simulink model "torque_structure"  (R2024b)
settings: Solver=FixedStepDiscrete  StartTime=0.0  StopTime=10.0  FixedStep=Ts  RelTol=1e-3
values from neighbouring files (symbols this model uses):
  g = 9.81    [main_data_vehicle.m]
  L = 1.55    [main_data_vehicle.m]
  lf = L*fr    (= 0.7905)    [main_data_vehicle.m]
  lr = L-lf    (= 0.7595)    [main_data_vehicle.m]
  Re = 0.259    [main_data_vehicle.m]
  TC = 1    [main_data_vehicle.m]
  TV = 1    [main_data_vehicle.m]
undefined symbols (not defined in the file or in its folder): DiscIntNeverNeededParam
libraries: simulink_extras x4, simulink x4, slpidlib x3
settings Model: Creator=marti  LastModifiedBy=marti

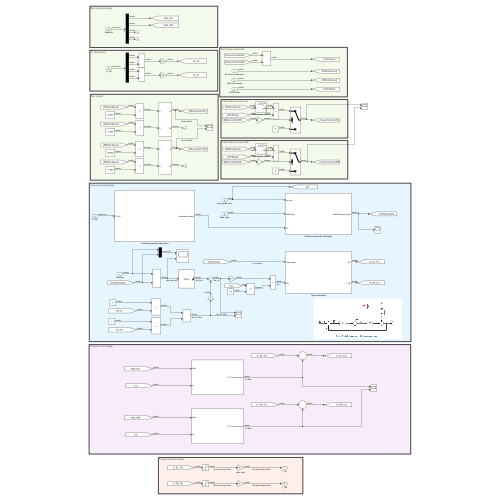
[thumbnail: Simulink's stored preview of the top-level diagram]
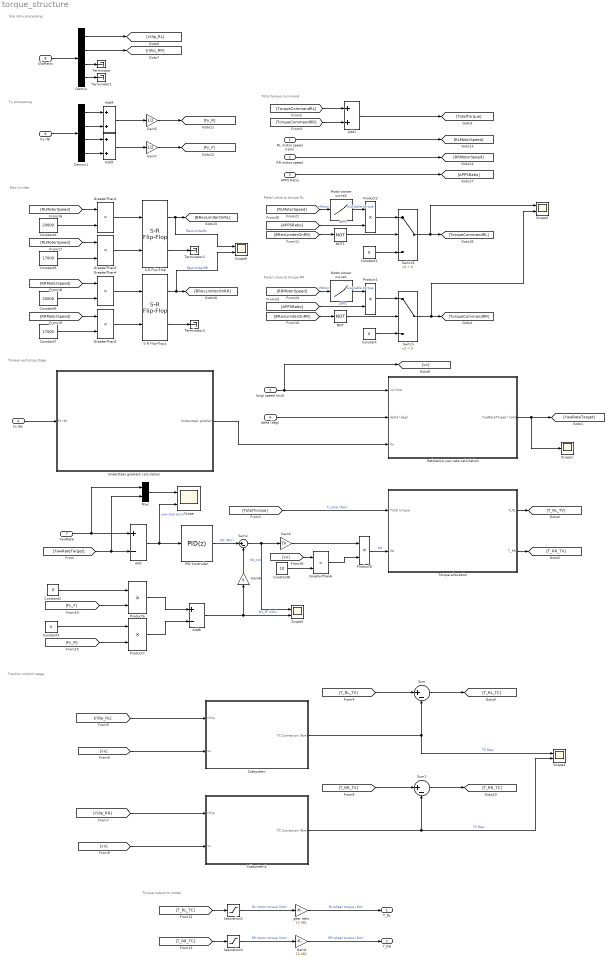
== system torque_structure ==
  note: Rev Limiter
  note: Fy processing
  note: Torque output to model
  note: Traction control stage
  note: Slip ratio processing
  note: Torque vectoring stage
  note: Total torque command
  note: Pedal value to torque RL
  note: Pedal value to torque RR
  RL motor speed (rpm) : Inport
  RR motor speed : Inport  Port=2
  APPS Ratio : Inport  Port=3
  Fz (N) : Inport  Port=4
  longi speed (m/s) : Inport  Port=5
  delta (deg) : Inport  Port=6
  YawRate : Inport  Port=7
  SlipRatio : Inport  Port=8
  Fy (N) : Inport  Port=9
  Add : Sum  Inputs=+-
  Add1 : Sum
  Add4 : Sum
  Add5 : Sum
  Add6 : Sum  Inputs=+-
  Constant : Constant  Value=0
  Constant1 : Constant  Value=0
  Constant2 : Constant  Value=lf
  Constant3 : Constant  Value=lr
  Constant4 : Constant  Value=20000
  Constant5 : Constant  Value=17000
  Constant6 : Constant  Value=20000
  Constant7 : Constant  Value=17000
  Constant8 : Constant  Value=10
  Demux : Demux
  Demux1 : Demux
  Gain2 : Gain  Gain=TV
  Gain5 : Gain  Gain=1/2
  Gain6 : Gain  Gain=12.481
  Gain7 : Gain  Gain=1/2
  Gain8 : Gain  Gain=0
  GreaterThan2 : RelationalOperator  Operator=>  OutDataTypeStr=boolean  RndMeth=Simplest  InputSameDT=off
  GreaterThan3 : RelationalOperator  Operator=<  OutDataTypeStr=boolean  RndMeth=Simplest  InputSameDT=off
  GreaterThan4 : RelationalOperator  Operator=>  OutDataTypeStr=boolean  RndMeth=Simplest  InputSameDT=off
  GreaterThan5 : RelationalOperator  Operator=<  OutDataTypeStr=boolean  RndMeth=Simplest  InputSameDT=off
  GreaterThan6 : RelationalOperator  Operator=>  OutDataTypeStr=boolean  RndMeth=Simplest  InputSameDT=off
  Motor power curve1 : Lookup_n-D  NumberOfTableDimensions=1  BreakpointsForDimension1=[0 11500 20000 20001]  Table=[32 32 18 0]  ExtrapMethod=Clip  UseLastTableValue=on  InternalRulePriority=Speed  RndMeth=Simplest
  Motor power curve2 : Lookup_n-D  NumberOfTableDimensions=1  BreakpointsForDimension1=[0 11500 20000 20001]  Table=[32 32 18 0]  ExtrapMethod=Clip  UseLastTableValue=on  InternalRulePriority=Speed  RndMeth=Simplest
  Mux : Mux  Inputs=2
  NOT : Logic  Operator=NOT  IconShape=distinctive  AllPortsSameDT=off  OutDataTypeStr=boolean
  NOT1 : Logic  Operator=NOT  IconShape=distinctive  AllPortsSameDT=off  OutDataTypeStr=boolean
  PID Controller : slpidlib/PID Controller  Controller=PID  Form=Parallel  TimeDomain=Discrete-time  UseExternalTs=off  SampleTime=-1  IntegratorMethod=Forward Euler  FilterMethod=Forward Euler  ControllerParametersSource=internal  P=100  I=0  UseKiTs=off  D=0  UseExternalDerivativeSource=off  N=100  UseFilter=on  TunerSelectOption=Transfer Function Based (PID Tuner App)  InitialConditionSource=internal  InitialConditionForIntegrator=0  InitialConditionForFilter=0  DifferentiatorICPrevScaledInput=0  ExternalReset=none  TrackingMode=off  Kt=1  LimitOutput=on  SatLimitsSource=internal  UpperSaturationLimit=500  LowerSaturationLimit=-500  LinearizeAsGain=on  AntiWindupMode=clamping  Kb=10  LimitIntegrator=off  UpperIntegratorSaturationLimit=inf  LowerIntegratorSaturationLimit=-inf  POutMin=[]  POutMax=[]  IOutMin=[]  IOutMax=[]  DOutMin=[]  DOutMax=[]  NOutMin=[]  NOutMax=[]  SumOutMin=[]  SumOutMax=[]  SaturationOutMin=[]  SaturationOutMax=[]  PParamMin=[]  PParamMax=[]  IParamMin=[]  IParamMax=[]  DParamMin=[]  DParamMax=[]  NParamMin=[]  NParamMax=[]  KbParamMin=[]  KbParamMax=[]  KtParamMin=[]  KtParamMax=[]  KbOutMin=[]  KbOutMax=[]  KtOutMin=[]  KtOutMax=[]  IntegratorOutMin=[]  IntegratorOutMax=[]  FilterOutMin=[]  FilterOutMax=[]  SumI1OutMin=[]  SumI1OutMax=[]  SumI2OutMin=[]  SumI2OutMax=[]  SumI3OutMin=[]  SumI3OutMax=[]  SumI4OutMin=[]  SumI4OutMax=[]  SumDOutMin=[]  SumDOutMax=[]  DifferentiatorOutMin=[]  DifferentiatorOutMax=[]  FilterDiffOutCoefMin=[]  FilterDiffOutCoefMax=[]  ReciprocalOutMin=[]  ReciprocalOutMax=[]  SumDenOutMin=[]  SumDenOutMax=[]  SumNumOutMin=[]  SumNumOutMax=[]  DivideOutMin=[]  DivideOutMax=[]  UdiffTsProdOutMin=[]  UdiffTsProdOutMax=[]  NTsProdOutMin=[]  NTsProdOutMax=[]  UintegralTsProdOutMin=[]  UintegralTsProdOutMax=[]  UngainTsProdOutMin=[]  UngainTsProdOutMax=[]  ClampingZeroOutDataTypeStr=Inherit: Inherit via back propagation  ClampingZeroOutMin=[]  ClampingZeroOutMax=[]  FilterDenConstantOutDataTypeStr=Inherit: Inherit via back propagation  FilterDenConstantOutMin=[]  FilterDenConstantOutMax=[]  PCopyOutDataTypeStr=Inherit: Inherit via back propagation  PCopyOutMin=[]  PCopyOutMax=[]  NCopyOutDataTypeStr=Inherit: Inherit via back propagation  NCopyOutMin=[]  NCopyOutMax=[]  IntegratorContinuousStateAttributes=''  IntegratorStateMustResolveToSignalObject=off  IntegratorRTWStateStorageClass=Auto  FilterContinuousStateAttributes=''  FilterStateMustResolveToSignalObject=off  FilterRTWStateStorageClass=Auto  ParallelPVariant=InternalParameters  IdealPVariant=Disabled  IVariant=InternalParameters  DVariant=InternalParameters  IntegratorVariant=Discrete  SatVariant=Enabled  AWVariant=DiscClampingParallel  PCopyVariant=Disabled  TRVariant=Disabled  FdbkBlocksVariant=Forward  IdealPFdbkVariant=Disabled  SatFdbkVariant=Disabled  DerivativeFilterVariant=ForwardEulerFilter  NVariant=InternalParameters  NCopyVariant=Disabled  FilterICVariant=InternalICsFilter  IntegratorICVariant=InternalICs  ExternalResetVariant=Disabled  TRSumVariant=Passthrough  SumFdbkVariant=Disabled  SumVariant=Sum_PID  TsampFilterVariant=InternalTs  TsampNgainVariant=Passthrough  TsampIntegralVariant=Disabled_SignalSpec  ExternalSaturationOutDataTypeStr=Inherit: Same as second input  DerivativeSourceVariant=ErrorSignal  PreIntVariant=InternalPreInt
  Product{1..2,6..8} (5 alike) : Product
  Reference yaw rate calculation : Subsystem
  S-R Flip-Flop : simulink_extras/Flip Flops/S-R Flip-Flop  initial_condition=0
  S-R Flip-Flop1 : simulink_extras/Flip Flops/S-R Flip-Flop  initial_condition=0
  Saturation2 : Saturate  UpperLimit=32  LowerLimit=-32
  Saturation3 : Saturate  UpperLimit=32  LowerLimit=-32
  Scope{,2..5} (5 alike) : Scope  NumInputPorts=2
  Scope1 : Scope
  Subsystem : Subsystem
  Subsystem1 : Subsystem
  Sum : Sum  Inputs=|+-
  Sum1 : Sum  Inputs=|+-
  Sum2 : Sum  Inputs=|+-
  Switch : Switch  Criteria=u2 > Threshold  SaturateOnIntegerOverflow=off  InputSameDT=off
  Switch1 : Switch  Criteria=u2 > Threshold  SaturateOnIntegerOverflow=off  InputSameDT=off
  Terminator{,1..3} (4 alike) : Terminator
  Torque allocation : Subsystem
  Understeer gradient calculation : Subsystem
  gear ratio : Gain  Gain=12.481
  T_RL : Outport
  T_RR : Outport  Port=2
  wires:
  Fz (N)/1 -> Understeer gradient calculation/1(Fz (N))
  Understeer gradient calculation/1(Understeer gradient) -> Reference yaw rate calculation/3(Ku)
  delta (deg)/1 -> Reference yaw rate calculation/2(delta (deg))
  longi speed (m/s)/1 -> [vx], Reference yaw rate calculation/1(vx (m/s))
  Reference yaw rate calculation/1(YawRateTarget (rad/s)) -> Scope1/1, [YawRateTarget]
  YawRate/1 -> Mux/1, Add/1
  [YawRateTarget] -> Mux/2, Add/2
  Add/1 -> Scope/2, PID Controller/1  "yaw rate error"
  [TotalTorque] -> Torque allocation/1(Total torque)  "T_total (Nm)"
  [TorqueCommandRL] -> Add1/1
  [TorqueCommandRR] -> Add1/2
  Add1/1 -> [TotalTorque]
  Torque allocation/1(T_RL) -> [T_RL_TV]
  Torque allocation/2(T_RR) -> [T_RR_TV]
  SlipRatio/1 -> Demux/1
  Demux/1 -> [rSlip_RL]
  Demux/2 -> [rSlip_RR]
  Demux/3 -> Terminator/1
  Demux/4 -> Terminator1/1
  [T_RL_TV] -> Sum/1
  [T_RR_TV] -> Sum1/1
  [T_RL_TC] -> Saturation2/1
  [T_RR_TC] -> Saturation3/1
  Saturation2/1 -> gear ratio/1  "RL motor torque (Nm)"
  Saturation3/1 -> Gain6/1  "RR motor torque (Nm)"
  gear ratio/1 -> T_RL/1  "RL wheel torque (Nm)"
  Gain6/1 -> T_RR/1  "RR wheel torque (Nm)"
  Sum/1 -> [T_RL_TC]
  Sum1/1 -> [T_RR_TC]
  Mux/1 -> Scope/1
  Fy (N)/1 -> Demux1/1
  Demux1/1 -> Add4/1
  Demux1/2 -> Add4/2
  Demux1/3 -> Add5/1
  Demux1/4 -> Add5/2
  Add4/1 -> Gain5/1
  Add5/1 -> Gain7/1
  Gain5/1 -> [Fy_R]
  Gain7/1 -> [Fy_F]
  Constant2/1 -> Product6/1
  [Fy_F] -> Product6/2
  [Fy_R] -> Product7/2
  Constant3/1 -> Product7/1
  Product6/1 -> Add6/1
  Product7/1 -> Add6/2
  PID Controller/1 -> Sum2/1  "Mz (Nm)"
  Sum2/1 -> Scope2/1, Gain2/1  "Mz_tot"
  Add6/1 -> Gain8/1, Scope2/2  "Mz_FF (Nm)"
  RL motor speed (rpm)/1 -> [RLMotorSpeed]
  RR motor speed/1 -> [RRMotorSpeed]
  [RLMotorSpeed] -> GreaterThan2/1
  Constant4/1 -> GreaterThan2/2
  GreaterThan2/1 -> S-R Flip-Flop/1
  Constant5/1 -> GreaterThan3/2
  [RLMotorSpeed] -> GreaterThan3/1
  GreaterThan3/1 -> S-R Flip-Flop/2
  S-R Flip-Flop/1 -> Scope5/1, [BRevLimiterOnRL]  "RevLimiterRL"
  S-R Flip-Flop/2 -> Terminator2/1
  S-R Flip-Flop1/2 -> Terminator3/1
  S-R Flip-Flop1/1 -> Scope5/2, [BRevLimiterOnRR]  "RevLimiterRR"
  GreaterThan5/1 -> S-R Flip-Flop1/2
  [RRMotorSpeed] -> GreaterThan5/1
  Constant7/1 -> GreaterThan5/2
  GreaterThan4/1 -> S-R Flip-Flop1/1
  Constant6/1 -> GreaterThan4/2
  [RRMotorSpeed] -> GreaterThan4/1
  APPS Ratio/1 -> [APPSRatio]
  [APPSRatio] -> Product1/2  "APPS"
  Motor power curve1/1 -> Product1/1  "available torque"
  [RRMotorSpeed] -> Motor power curve1/1  "nMotor"
  [vx] -> GreaterThan6/1
  Product8/1 -> Torque allocation/2(Mz)  "Mz"
  Gain2/1 -> Product8/1
  Gain8/1 -> Sum2/2
  Constant8/1 -> GreaterThan6/2
  GreaterThan6/1 -> Product8/2
  [rSlip_RL] -> Subsystem/1(rSlip)
  [vx] -> Subsystem/2(vx)
  [vx] -> Subsystem1/2(vx)
  [rSlip_RR] -> Subsystem1/1(rSlip)
  Switch/1 -> Scope3/2, [TorqueCommandRR]
  Product1/1 -> Switch/1
  [BRevLimiterOnRR] -> NOT/1
  NOT/1 -> Switch/2
  Constant/1 -> Switch/3
  Constant1/1 -> Switch1/3
  NOT1/1 -> Switch1/2
  [BRevLimiterOnRR] -> NOT1/1
  Product2/1 -> Switch1/1
  Switch1/1 -> Scope3/1, [TorqueCommandRL]
  [RLMotorSpeed] -> Motor power curve2/1  "nMotor"
  Motor power curve2/1 -> Product2/1  "available torque"
  [APPSRatio] -> Product2/2  "APPS"
  Subsystem/1(TC Correction (Nm)) -> Scope4/1, Sum/2  "TC Raw"
  Subsystem1/1(TC Correction (Nm)) -> Scope4/2, Sum1/2  "TC Raw"

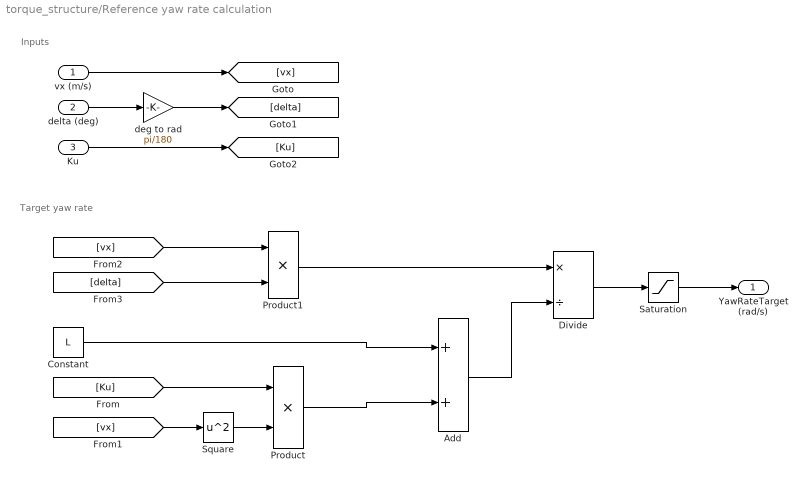
== system torque_structure/Reference yaw rate calculation ==
  note: Target yaw rate
  note: Inputs
  vx (m/s) : Inport
  delta (deg) : Inport  Port=2
  Ku : Inport  Port=3
  Add : Sum
  Constant : Constant  Value=L
  Divide : Product  Inputs=*/
  Product : Product
  Product1 : Product
  Saturation : Saturate  UpperLimit=1.5  LowerLimit=-1.5
  Square : Math  Operator=square
  deg to rad : Gain  Gain=pi/180
  YawRateTarget (rad/s) : Outport
  wires:
  vx (m/s)/1 -> [vx]
  delta (deg)/1 -> deg to rad/1
  deg to rad/1 -> [delta]
  Ku/1 -> [Ku]
  [vx] -> Square/1
  Square/1 -> Product/2
  [Ku] -> Product/1
  Product/1 -> Add/2
  Constant/1 -> Add/1
  [vx] -> Product1/1
  [delta] -> Product1/2
  Product1/1 -> Divide/1
  Add/1 -> Divide/2
  Divide/1 -> Saturation/1
  Saturation/1 -> YawRateTarget (rad/s)/1

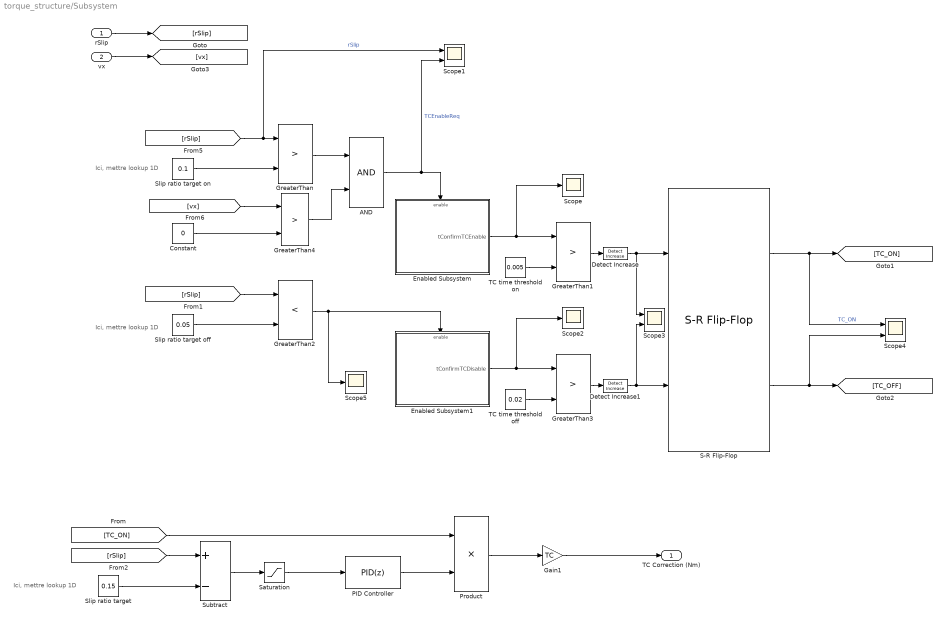
== system torque_structure/Subsystem ==
  note: Ici, mettre lookup 1D
  note: Ici, mettre lookup 1D
  note: Ici, mettre lookup 1D
  rSlip : Inport
  vx : Inport  Port=2
  AND : Logic  AllPortsSameDT=off  OutDataTypeStr=boolean
  Constant : Constant  Value=0
  Detect Increase : simulink/Logic and Bit Operations/Detect Increase  vinit=0.0  OutDataTypeStr=boolean
  Detect Increase1 : simulink/Logic and Bit Operations/Detect Increase  vinit=0.0  OutDataTypeStr=boolean
  Enabled Subsystem : Subsystem  TreatAsAtomicUnit=on
  Enabled Subsystem1 : Subsystem  TreatAsAtomicUnit=on
  Gain1 : Gain  Gain=TC
  GreaterThan{,1,3..4} (4 alike) : RelationalOperator  Operator=>  OutDataTypeStr=boolean  RndMeth=Simplest  InputSameDT=off
  GreaterThan2 : RelationalOperator  Operator=<  OutDataTypeStr=boolean  RndMeth=Simplest  InputSameDT=off
  PID Controller : slpidlib/PID Controller  Controller=PID  Form=Parallel  TimeDomain=Discrete-time  UseExternalTs=off  SampleTime=-1  IntegratorMethod=Forward Euler  FilterMethod=Forward Euler  ControllerParametersSource=internal  P=100  I=20  UseKiTs=off  D=0  UseExternalDerivativeSource=off  N=100  UseFilter=on  TunerSelectOption=Transfer Function Based (PID Tuner App)  InitialConditionSource=internal  InitialConditionForIntegrator=0  InitialConditionForFilter=0  DifferentiatorICPrevScaledInput=0  ExternalReset=none  TrackingMode=off  Kt=1  LimitOutput=on  SatLimitsSource=internal  UpperSaturationLimit=30  LowerSaturationLimit=0  LinearizeAsGain=on  AntiWindupMode=clamping  Kb=1  LimitIntegrator=off  UpperIntegratorSaturationLimit=inf  LowerIntegratorSaturationLimit=-inf  POutMin=[]  POutMax=[]  IOutMin=[]  IOutMax=[]  DOutMin=[]  DOutMax=[]  NOutMin=[]  NOutMax=[]  SumOutMin=[]  SumOutMax=[]  SaturationOutMin=[]  SaturationOutMax=[]  PParamMin=[]  PParamMax=[]  IParamMin=[]  IParamMax=[]  DParamMin=[]  DParamMax=[]  NParamMin=[]  NParamMax=[]  KbParamMin=[]  KbParamMax=[]  KtParamMin=[]  KtParamMax=[]  KbOutMin=[]  KbOutMax=[]  KtOutMin=[]  KtOutMax=[]  IntegratorOutMin=[]  IntegratorOutMax=[]  FilterOutMin=[]  FilterOutMax=[]  SumI1OutMin=[]  SumI1OutMax=[]  SumI2OutMin=[]  SumI2OutMax=[]  SumI3OutMin=[]  SumI3OutMax=[]  SumI4OutMin=[]  SumI4OutMax=[]  SumDOutMin=[]  SumDOutMax=[]  DifferentiatorOutMin=[]  DifferentiatorOutMax=[]  FilterDiffOutCoefMin=[]  FilterDiffOutCoefMax=[]  ReciprocalOutMin=[]  ReciprocalOutMax=[]  SumDenOutMin=[]  SumDenOutMax=[]  SumNumOutMin=[]  SumNumOutMax=[]  DivideOutMin=[]  DivideOutMax=[]  UdiffTsProdOutMin=[]  UdiffTsProdOutMax=[]  NTsProdOutMin=[]  NTsProdOutMax=[]  UintegralTsProdOutMin=[]  UintegralTsProdOutMax=[]  UngainTsProdOutMin=[]  UngainTsProdOutMax=[]  ClampingZeroOutDataTypeStr=Inherit: Inherit via back propagation  ClampingZeroOutMin=[]  ClampingZeroOutMax=[]  FilterDenConstantOutDataTypeStr=Inherit: Inherit via back propagation  FilterDenConstantOutMin=[]  FilterDenConstantOutMax=[]  PCopyOutDataTypeStr=Inherit: Inherit via back propagation  PCopyOutMin=[]  PCopyOutMax=[]  NCopyOutDataTypeStr=Inherit: Inherit via back propagation  NCopyOutMin=[]  NCopyOutMax=[]  IntegratorContinuousStateAttributes=''  IntegratorStateMustResolveToSignalObject=off  IntegratorRTWStateStorageClass=Auto  FilterContinuousStateAttributes=''  FilterStateMustResolveToSignalObject=off  FilterRTWStateStorageClass=Auto  ParallelPVariant=InternalParameters  IdealPVariant=Disabled  IVariant=InternalParameters  DVariant=InternalParameters  IntegratorVariant=Discrete  SatVariant=Enabled  AWVariant=DiscClampingParallel  PCopyVariant=Disabled  TRVariant=Disabled  FdbkBlocksVariant=Forward  IdealPFdbkVariant=Disabled  SatFdbkVariant=Disabled  DerivativeFilterVariant=ForwardEulerFilter  NVariant=InternalParameters  NCopyVariant=Disabled  FilterICVariant=InternalICsFilter  IntegratorICVariant=InternalICs  ExternalResetVariant=Disabled  TRSumVariant=Passthrough  SumFdbkVariant=Disabled  SumVariant=Sum_PID  TsampFilterVariant=InternalTs  TsampNgainVariant=Passthrough  TsampIntegralVariant=Disabled_SignalSpec  ExternalSaturationOutDataTypeStr=Inherit: Same as second input  DerivativeSourceVariant=ErrorSignal  PreIntVariant=InternalPreInt
  Product : Product
  S-R Flip-Flop : simulink_extras/Flip Flops/S-R Flip-Flop  initial_condition=0
  Saturation : Saturate  UpperLimit=1  LowerLimit=0
  Scope : Scope
  Scope1 : Scope  NumInputPorts=2
  Scope2 : Scope
  Scope3 : Scope  NumInputPorts=2
  Scope4 : Scope  NumInputPorts=2
  Scope5 : Scope
  Slip ratio target : Constant  Value=0.15
  Slip ratio target off : Constant  Value=0.05
  Slip ratio target on : Constant  Value=0.1
  Subtract : Sum  Inputs=+-
  TC time threshold off : Constant  Value=0.02
  TC time threshold on : Constant  Value=0.005
  TC Correction (Nm) : Outport
  wires:
  Slip ratio target/1 -> Subtract/2
  [TC_ON] -> Product/1
  Slip ratio target off/1 -> GreaterThan2/2
  S-R Flip-Flop/1 -> Scope4/1, [TC_ON]  "TC_ON"
  [rSlip] -> Subtract/1
  GreaterThan1/1 -> Detect Increase/1
  Slip ratio target on/1 -> GreaterThan/2
  Saturation/1 -> PID Controller/1
  S-R Flip-Flop/2 -> Scope4/2, [TC_OFF]
  GreaterThan4/1 -> AND/2
  TC time threshold off/1 -> GreaterThan3/2
  [rSlip] -> Scope1/1, GreaterThan/1  "rSlip"
  Enabled Subsystem/1(tConfirmTCEnable) -> GreaterThan1/1, Scope/1
  Subtract/1 -> Saturation/1
  [vx] -> GreaterThan4/1
  Constant/1 -> GreaterThan4/2
  Enabled Subsystem1/1(tConfirmTCDisable) -> Scope2/1, GreaterThan3/1
  GreaterThan/1 -> AND/1
  Product/1 -> Gain1/1
  vx/1 -> [vx]
  Gain1/1 -> TC Correction (Nm)/1
  GreaterThan3/1 -> Detect Increase1/1
  TC time threshold on/1 -> GreaterThan1/2
  [rSlip] -> GreaterThan2/1
  rSlip/1 -> [rSlip]
  AND/1 -> Scope1/2, Enabled Subsystem/Enable  "TCEnableReq"
  PID Controller/1 -> Product/2
  GreaterThan2/1 -> Scope5/1, Enabled Subsystem1/Enable
  Detect Increase/1 -> Scope3/1, S-R Flip-Flop/1
  Detect Increase1/1 -> Scope3/2, S-R Flip-Flop/2

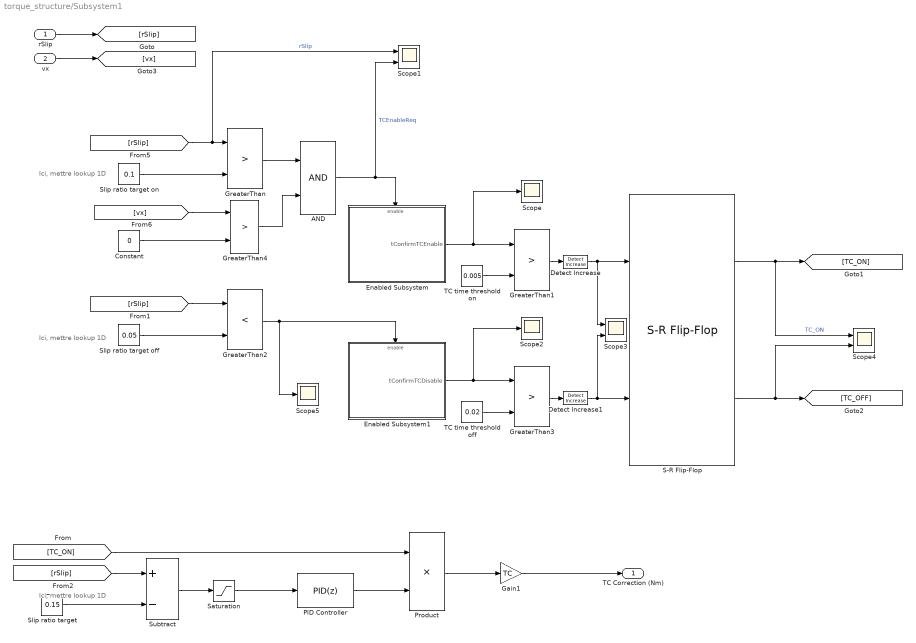
== system torque_structure/Subsystem1 ==
  note: Ici, mettre lookup 1D
  note: Ici, mettre lookup 1D
  note: Ici, mettre lookup 1D
  rSlip : Inport
  vx : Inport  Port=2
  AND : Logic  AllPortsSameDT=off  OutDataTypeStr=boolean
  Constant : Constant  Value=0
  Detect Increase : simulink/Logic and Bit Operations/Detect Increase  vinit=0.0  OutDataTypeStr=boolean
  Detect Increase1 : simulink/Logic and Bit Operations/Detect Increase  vinit=0.0  OutDataTypeStr=boolean
  Enabled Subsystem : Subsystem  TreatAsAtomicUnit=on
  Enabled Subsystem1 : Subsystem  TreatAsAtomicUnit=on
  Gain1 : Gain  Gain=TC
  GreaterThan{,1,3..4} (4 alike) : RelationalOperator  Operator=>  OutDataTypeStr=boolean  RndMeth=Simplest  InputSameDT=off
  GreaterThan2 : RelationalOperator  Operator=<  OutDataTypeStr=boolean  RndMeth=Simplest  InputSameDT=off
  PID Controller : slpidlib/PID Controller  Controller=PID  Form=Parallel  TimeDomain=Discrete-time  UseExternalTs=off  SampleTime=-1  IntegratorMethod=Forward Euler  FilterMethod=Forward Euler  ControllerParametersSource=internal  P=100  I=20  UseKiTs=off  D=0  UseExternalDerivativeSource=off  N=100  UseFilter=on  TunerSelectOption=Transfer Function Based (PID Tuner App)  InitialConditionSource=internal  InitialConditionForIntegrator=0  InitialConditionForFilter=0  DifferentiatorICPrevScaledInput=0  ExternalReset=none  TrackingMode=off  Kt=1  LimitOutput=on  SatLimitsSource=internal  UpperSaturationLimit=30  LowerSaturationLimit=0  LinearizeAsGain=on  AntiWindupMode=clamping  Kb=1  LimitIntegrator=off  UpperIntegratorSaturationLimit=inf  LowerIntegratorSaturationLimit=-inf  POutMin=[]  POutMax=[]  IOutMin=[]  IOutMax=[]  DOutMin=[]  DOutMax=[]  NOutMin=[]  NOutMax=[]  SumOutMin=[]  SumOutMax=[]  SaturationOutMin=[]  SaturationOutMax=[]  PParamMin=[]  PParamMax=[]  IParamMin=[]  IParamMax=[]  DParamMin=[]  DParamMax=[]  NParamMin=[]  NParamMax=[]  KbParamMin=[]  KbParamMax=[]  KtParamMin=[]  KtParamMax=[]  KbOutMin=[]  KbOutMax=[]  KtOutMin=[]  KtOutMax=[]  IntegratorOutMin=[]  IntegratorOutMax=[]  FilterOutMin=[]  FilterOutMax=[]  SumI1OutMin=[]  SumI1OutMax=[]  SumI2OutMin=[]  SumI2OutMax=[]  SumI3OutMin=[]  SumI3OutMax=[]  SumI4OutMin=[]  SumI4OutMax=[]  SumDOutMin=[]  SumDOutMax=[]  DifferentiatorOutMin=[]  DifferentiatorOutMax=[]  FilterDiffOutCoefMin=[]  FilterDiffOutCoefMax=[]  ReciprocalOutMin=[]  ReciprocalOutMax=[]  SumDenOutMin=[]  SumDenOutMax=[]  SumNumOutMin=[]  SumNumOutMax=[]  DivideOutMin=[]  DivideOutMax=[]  UdiffTsProdOutMin=[]  UdiffTsProdOutMax=[]  NTsProdOutMin=[]  NTsProdOutMax=[]  UintegralTsProdOutMin=[]  UintegralTsProdOutMax=[]  UngainTsProdOutMin=[]  UngainTsProdOutMax=[]  ClampingZeroOutDataTypeStr=Inherit: Inherit via back propagation  ClampingZeroOutMin=[]  ClampingZeroOutMax=[]  FilterDenConstantOutDataTypeStr=Inherit: Inherit via back propagation  FilterDenConstantOutMin=[]  FilterDenConstantOutMax=[]  PCopyOutDataTypeStr=Inherit: Inherit via back propagation  PCopyOutMin=[]  PCopyOutMax=[]  NCopyOutDataTypeStr=Inherit: Inherit via back propagation  NCopyOutMin=[]  NCopyOutMax=[]  IntegratorContinuousStateAttributes=''  IntegratorStateMustResolveToSignalObject=off  IntegratorRTWStateStorageClass=Auto  FilterContinuousStateAttributes=''  FilterStateMustResolveToSignalObject=off  FilterRTWStateStorageClass=Auto  ParallelPVariant=InternalParameters  IdealPVariant=Disabled  IVariant=InternalParameters  DVariant=InternalParameters  IntegratorVariant=Discrete  SatVariant=Enabled  AWVariant=DiscClampingParallel  PCopyVariant=Disabled  TRVariant=Disabled  FdbkBlocksVariant=Forward  IdealPFdbkVariant=Disabled  SatFdbkVariant=Disabled  DerivativeFilterVariant=ForwardEulerFilter  NVariant=InternalParameters  NCopyVariant=Disabled  FilterICVariant=InternalICsFilter  IntegratorICVariant=InternalICs  ExternalResetVariant=Disabled  TRSumVariant=Passthrough  SumFdbkVariant=Disabled  SumVariant=Sum_PID  TsampFilterVariant=InternalTs  TsampNgainVariant=Passthrough  TsampIntegralVariant=Disabled_SignalSpec  ExternalSaturationOutDataTypeStr=Inherit: Same as second input  DerivativeSourceVariant=ErrorSignal  PreIntVariant=InternalPreInt
  Product : Product
  S-R Flip-Flop : simulink_extras/Flip Flops/S-R Flip-Flop  initial_condition=0
  Saturation : Saturate  UpperLimit=1  LowerLimit=0
  Scope : Scope
  Scope1 : Scope  NumInputPorts=2
  Scope2 : Scope
  Scope3 : Scope  NumInputPorts=2
  Scope4 : Scope  NumInputPorts=2
  Scope5 : Scope
  Slip ratio target : Constant  Value=0.15
  Slip ratio target off : Constant  Value=0.05
  Slip ratio target on : Constant  Value=0.1
  Subtract : Sum  Inputs=+-
  TC time threshold off : Constant  Value=0.02
  TC time threshold on : Constant  Value=0.005
  TC Correction (Nm) : Outport
  wires:
  Detect Increase1/1 -> S-R Flip-Flop/2, Scope3/2
  Detect Increase/1 -> S-R Flip-Flop/1, Scope3/1
  GreaterThan2/1 -> Enabled Subsystem1/Enable, Scope5/1
  PID Controller/1 -> Product/2
  AND/1 -> Enabled Subsystem/Enable, Scope1/2  "TCEnableReq"
  rSlip/1 -> [rSlip]
  [rSlip] -> GreaterThan2/1
  TC time threshold on/1 -> GreaterThan1/2
  GreaterThan3/1 -> Detect Increase1/1
  Gain1/1 -> TC Correction (Nm)/1
  vx/1 -> [vx]
  Product/1 -> Gain1/1
  GreaterThan/1 -> AND/1
  Enabled Subsystem1/1(tConfirmTCDisable) -> GreaterThan3/1, Scope2/1
  Constant/1 -> GreaterThan4/2
  [vx] -> GreaterThan4/1
  Subtract/1 -> Saturation/1
  Enabled Subsystem/1(tConfirmTCEnable) -> Scope/1, GreaterThan1/1
  [rSlip] -> GreaterThan/1, Scope1/1  "rSlip"
  TC time threshold off/1 -> GreaterThan3/2
  GreaterThan4/1 -> AND/2
  S-R Flip-Flop/2 -> [TC_OFF], Scope4/2
  Saturation/1 -> PID Controller/1
  Slip ratio target on/1 -> GreaterThan/2
  GreaterThan1/1 -> Detect Increase/1
  [rSlip] -> Subtract/1
  S-R Flip-Flop/1 -> [TC_ON], Scope4/1  "TC_ON"
  Slip ratio target off/1 -> GreaterThan2/2
  [TC_ON] -> Product/1
  Slip ratio target/1 -> Subtract/2

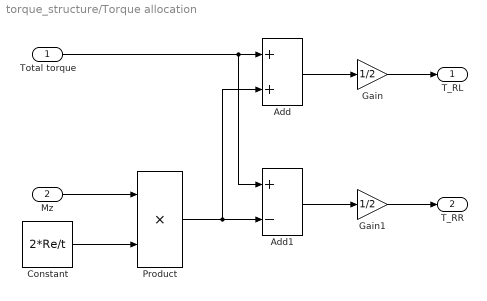
== system torque_structure/Torque allocation ==
  Total torque : Inport
  Mz : Inport  Port=2
  Add : Sum
  Add1 : Sum  Inputs=+-
  Constant : Constant  Value=2*Re/t
  Gain : Gain  Gain=1/2
  Gain1 : Gain  Gain=1/2
  Product : Product
  T_RL : Outport
  T_RR : Outport  Port=2
  wires:
  Constant/1 -> Product/2
  Mz/1 -> Product/1
  Total torque/1 -> Add1/1, Add/1
  Product/1 -> Add1/2, Add/2
  Add/1 -> Gain/1
  Add1/1 -> Gain1/1
  Gain/1 -> T_RL/1
  Gain1/1 -> T_RR/1

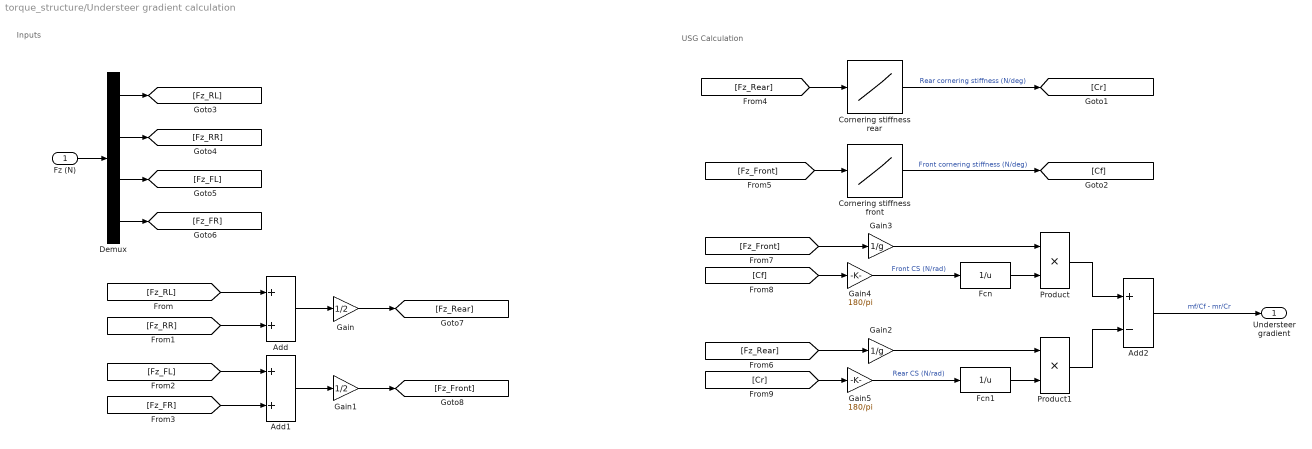
== system torque_structure/Understeer gradient calculation ==
  note: USG Calculation
  note: Inputs
  Fz (N) : Inport
  Add : Sum
  Add1 : Sum
  Add2 : Sum  Inputs=+-
  Cornering stiffness front : Lookup_n-D  NumberOfTableDimensions=1  BreakpointsForDimension1=[200 650 1450 1600]  Table=[64 286 496 520]  InternalRulePriority=Speed  RndMeth=Simplest
  Cornering stiffness rear : Lookup_n-D  NumberOfTableDimensions=1  BreakpointsForDimension1=[200 650 1450 1600]  Table=[64 286 496 520]  InternalRulePriority=Speed  RndMeth=Simplest
  Demux : Demux
  Fcn : Fcn  Expr=1/u
  Fcn1 : Fcn  Expr=1/u
  Gain : Gain  Gain=1/2
  Gain1 : Gain  Gain=1/2
  Gain2 : Gain  Gain=1/g
  Gain3 : Gain  Gain=1/g
  Gain4 : Gain  Gain=180/pi
  Gain5 : Gain  Gain=180/pi
  Product : Product
  Product1 : Product
  Understeer gradient : Outport
  wires:
  Demux/1 -> [Fz_RL]
  [Fz_Front] -> Cornering stiffness front/1
  Cornering stiffness rear/1 -> [Cr]  "Rear cornering stiffness (N/deg)"
  Demux/2 -> [Fz_RR]
  Fz (N)/1 -> Demux/1
  Cornering stiffness front/1 -> [Cf]  "Front cornering stiffness (N/deg)"
  Demux/3 -> [Fz_FL]
  [Fz_Rear] -> Cornering stiffness rear/1
  Demux/4 -> [Fz_FR]
  [Fz_RL] -> Add/1
  [Fz_RR] -> Add/2
  Add/1 -> Gain/1
  Gain/1 -> [Fz_Rear]
  Gain1/1 -> [Fz_Front]
  Add1/1 -> Gain1/1
  [Fz_FR] -> Add1/2
  [Fz_FL] -> Add1/1
  [Fz_Front] -> Gain3/1
  Gain3/1 -> Product/1
  [Cf] -> Gain4/1
  [Cr] -> Gain5/1
  Gain2/1 -> Product1/1
  [Fz_Rear] -> Gain2/1
  Product/1 -> Add2/1
  Product1/1 -> Add2/2
  Add2/1 -> Understeer gradient/1  "mf/Cf - mr/Cr"
  Gain4/1 -> Fcn/1  "Front CS (N/rad)"
  Gain5/1 -> Fcn1/1  "Rear CS (N/rad)"
  Fcn/1 -> Product/2
  Fcn1/1 -> Product1/2

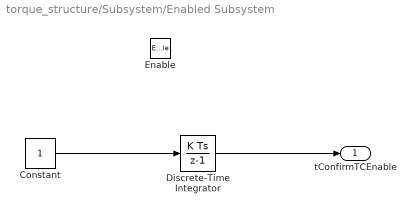
== system torque_structure/Subsystem/Enabled Subsystem ==
  Enable : EnablePort  StatesWhenEnabling=reset
  Constant : Constant
  Discrete-Time Integrator : DiscreteIntegrator  SampleTime=-1  ICPrevOutput=DiscIntNeverNeededParam  ICPrevScaledInput=DiscIntNeverNeededParam
  tConfirmTCEnable : Outport
  wires:
  Constant/1 -> Discrete-Time Integrator/1
  Discrete-Time Integrator/1 -> tConfirmTCEnable/1

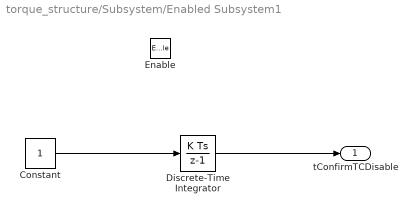
== system torque_structure/Subsystem/Enabled Subsystem1 ==
  Enable : EnablePort  StatesWhenEnabling=reset
  Constant : Constant
  Discrete-Time Integrator : DiscreteIntegrator  SampleTime=-1  ICPrevOutput=DiscIntNeverNeededParam  ICPrevScaledInput=DiscIntNeverNeededParam
  tConfirmTCDisable : Outport
  wires:
  Discrete-Time Integrator/1 -> tConfirmTCDisable/1
  Constant/1 -> Discrete-Time Integrator/1

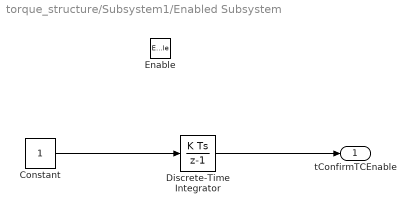
== system torque_structure/Subsystem1/Enabled Subsystem ==
  Enable : EnablePort  StatesWhenEnabling=reset
  Constant : Constant
  Discrete-Time Integrator : DiscreteIntegrator  SampleTime=-1  ICPrevOutput=DiscIntNeverNeededParam  ICPrevScaledInput=DiscIntNeverNeededParam
  tConfirmTCEnable : Outport
  wires:
  Discrete-Time Integrator/1 -> tConfirmTCEnable/1
  Constant/1 -> Discrete-Time Integrator/1

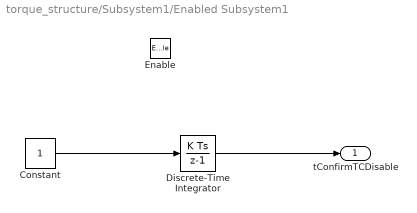
== system torque_structure/Subsystem1/Enabled Subsystem1 ==
  Enable : EnablePort  StatesWhenEnabling=reset
  Constant : Constant
  Discrete-Time Integrator : DiscreteIntegrator  SampleTime=-1  ICPrevOutput=DiscIntNeverNeededParam  ICPrevScaledInput=DiscIntNeverNeededParam
  tConfirmTCDisable : Outport
  wires:
  Constant/1 -> Discrete-Time Integrator/1
  Discrete-Time Integrator/1 -> tConfirmTCDisable/1
